simulink model "untitled"  (R2016a)
settings: Solver=VariableStepAuto  StartTime=0.0  StopTime=100  RelTol=1e-3
libraries: fuzblock x1, simulink x1
settings Model: Creator=Evand  LastModifiedBy=Evand

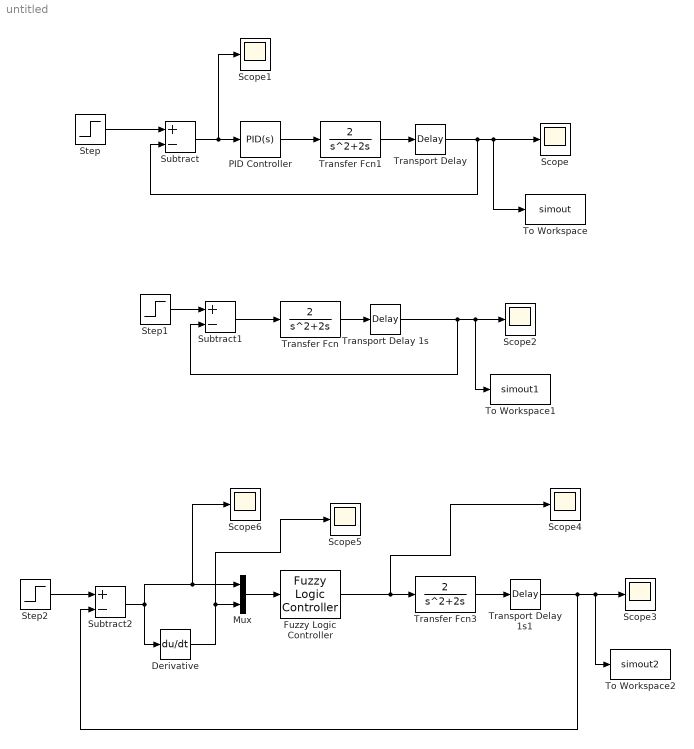
== system untitled ==
  Derivative : Derivative
  Fuzzy Logic Controller : fuzblock/Fuzzy Logic  Controller  fis='fuzzy.fis'
  Mux : Mux  Inputs=2
  PID Controller : simulink/Continuous/PID Controller  Controller=PID  TimeDomain=Continuous-time  SampleTime=-1  IntegratorMethod=Forward Euler  FilterMethod=Forward Euler  Form=Parallel  UseFilter=on  ControllerParametersSource=internal  P=0.8  I=0.1  D=1  N=100  InitialConditionSource=internal  InitialConditionForIntegrator=0  InitialConditionForFilter=0  ExternalReset=none  LimitOutput=off  UpperSaturationLimit=inf  LowerSaturationLimit=-inf  LinearizeAsGain=on  AntiWindupMode=none  Kb=1  TrackingMode=off  Kt=1  PParamMin=[]  PParamMax=[]  IParamMin=[]  IParamMax=[]  DParamMin=[]  DParamMax=[]  NParamMin=[]  NParamMax=[]  KbParamMin=[]  KbParamMax=[]  KtParamMin=[]  KtParamMax=[]  POutMin=[]  POutMax=[]  IOutMin=[]  IOutMax=[]  DOutMin=[]  DOutMax=[]  NOutMin=[]  NOutMax=[]  KbOutMin=[]  KbOutMax=[]  KtOutMin=[]  KtOutMax=[]  IntegratorOutMin=[]  IntegratorOutMax=[]  FilterOutMin=[]  FilterOutMax=[]  SumOutMin=[]  SumOutMax=[]  SumI1OutMin=[]  SumI1OutMax=[]  SumI2OutMin=[]  SumI2OutMax=[]  SumI3OutMin=[]  SumI3OutMax=[]  SumDOutMin=[]  SumDOutMax=[]  SaturationOutMin=[]  SaturationOutMax=[]  IntegratorContinuousStateAttributes=''  IntegratorStateMustResolveToSignalObject=off  IntegratorRTWStateStorageClass=Auto  FilterContinuousStateAttributes=''  FilterStateMustResolveToSignalObject=off  FilterRTWStateStorageClass=Auto  DifferentiatorICPrevScaledInput=0  DifferentiatorOutMin=[]  DifferentiatorOutMax=[]
  Scope{,1..6} (7 alike) : Scope
  Step : Step  Time=0  SampleTime=0
  Step1 : Step  Time=0  SampleTime=0
  Step2 : Step  Time=0  SampleTime=0
  Subtract : Sum  Inputs=+-
  Subtract1 : Sum  Inputs=+-
  Subtract2 : Sum  Inputs=+-
  To Workspace : ToWorkspace  VariableName=simout  SaveFormat=Timeseries  SampleTime=-1
  To Workspace1 : ToWorkspace  VariableName=simout1  SaveFormat=Timeseries  SampleTime=-1
  To Workspace2 : ToWorkspace  VariableName=simout2  SaveFormat=Timeseries  SampleTime=-1
  Transfer Fcn : TransferFcn  Numerator=[2]  Denominator=[1 2 0]
  Transfer Fcn1 : TransferFcn  Numerator=[2]  Denominator=[1 2 0]
  Transfer Fcn3 : TransferFcn  Numerator=[2]  Denominator=[1 2 0]
  Transport Delay : TransportDelay
  Transport Delay 1s : TransportDelay
  Transport Delay 1s1 : TransportDelay
  wires:
  Transfer Fcn/1 -> Transport Delay 1s/1
  Transport Delay 1s/1 -> Subtract1/2, To Workspace1/1, Scope2/1
  Step1/1 -> Subtract1/1
  Subtract1/1 -> Transfer Fcn/1
  Transfer Fcn1/1 -> Transport Delay/1
  Transport Delay/1 -> To Workspace/1, Scope/1, Subtract/2
  Step/1 -> Subtract/1
  Subtract/1 -> Scope1/1, PID Controller/1
  PID Controller/1 -> Transfer Fcn1/1
  Transfer Fcn3/1 -> Transport Delay 1s1/1
  Transport Delay 1s1/1 -> To Workspace2/1, Scope3/1, Subtract2/2
  Step2/1 -> Subtract2/1
  Subtract2/1 -> Derivative/1, Scope6/1, Mux/1
  Mux/1 -> Fuzzy Logic Controller/1
  Fuzzy Logic Controller/1 -> Scope4/1, Transfer Fcn3/1
  Derivative/1 -> Scope5/1, Mux/2
